simulink model "fadec_thermo_model"  (R2025b)
settings: Solver=FixedStepDiscrete  StartTime=0.0  StopTime=10.0  FixedStep=0.02  RelTol=1e-3

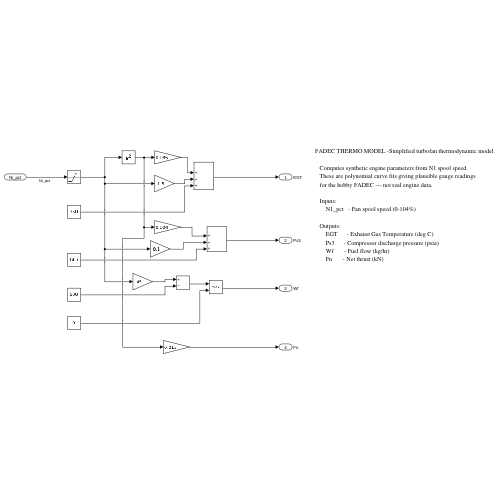
[thumbnail: Simulink's stored preview of the top-level diagram]
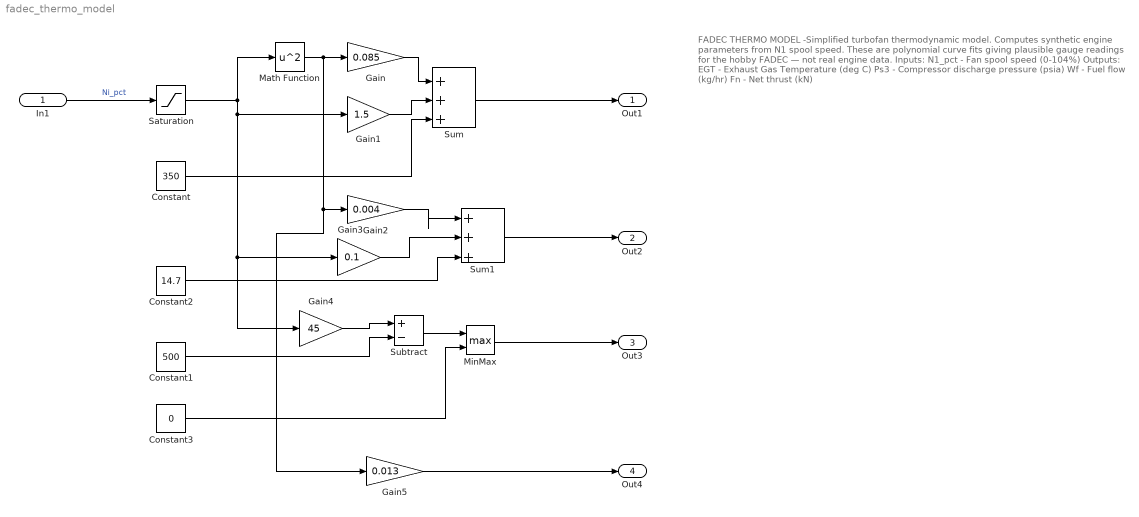
== system fadec_thermo_model ==
  note: FADEC THERMO MODEL -Simplified turbofan thermodynamic model.
      |
      |    Computes synthetic engine parameters from N1 spool speed.
      |    These are polynomial curve fits giving plausible gauge readings
      |    for the hobby FADEC — not real engine data.
      |
      |    Inputs:
      |        N1_pct   - Fan spool speed (0-104%)
      |
      |    Outputs:
      |        EGT      - Exhaust Gas Temperature (deg C)
      |        Ps3      - Compressor discharge pressure (psia)
      |        Wf       - Fuel flow (kg/hr)
      |        Fn       - Net thrust (kN)
  In1 : Inport
  Constant : Constant  Value=350
  Constant1 : Constant  Value=500
  Constant2 : Constant  Value=14.7
  Constant3 : Constant  Value=0
  Gain : Gain  Gain=0.085
  Gain1 : Gain  Gain=1.5
  Gain2 : Gain  Gain=0.004
  Gain3 : Gain  Gain=0.1
  Gain4 : Gain  Gain=45
  Gain5 : Gain  Gain=0.013
  Math Function : Math  Operator=square
  MinMax : MinMax  Function=max  Inputs=2
  Saturation : Saturate  UpperLimit=104  LowerLimit=0
  Subtract : Sum  Inputs=+-
  Sum : Sum  Inputs=|+++
  Sum1 : Sum  Inputs=|+++
  Out1 : Outport  SignalName=EGT
  Out2 : Outport  Port=2  SignalName=Ps3
  Out3 : Outport  Port=3  SignalName=Wf
  Out4 : Outport  Port=4  SignalName=Fn
  wires:
  In1/1 -> Saturation/1  "Ni_pct"
  Saturation/1 -> Math Function/1, Gain4/1, Gain3/1, Gain1/1
  Math Function/1 -> Gain5/1, Gain2/1, Gain/1
  Gain/1 -> Sum/1
  Gain1/1 -> Sum/2
  Constant/1 -> Sum/3
  Sum/1 -> Out1/1
  Gain2/1 -> Sum1/1
  Gain3/1 -> Sum1/2
  Constant2/1 -> Sum1/3
  Sum1/1 -> Out2/1
  Gain4/1 -> Subtract/1
  Constant1/1 -> Subtract/2
  Subtract/1 -> MinMax/1
  Constant3/1 -> MinMax/2
  MinMax/1 -> Out3/1
  Gain5/1 -> Out4/1
